simulink model "SqaureKF"  (Simulink 7.6)
settings: Solver=ode8  StartTime=0.0  StopTime=inf  FixedStep=0.01  RelTol=1e-3
libraries: aerolibanimutils x1, dspadpt3 x1, simulink x1
settings Model: Creator=Owen  LastModifiedBy=Owen

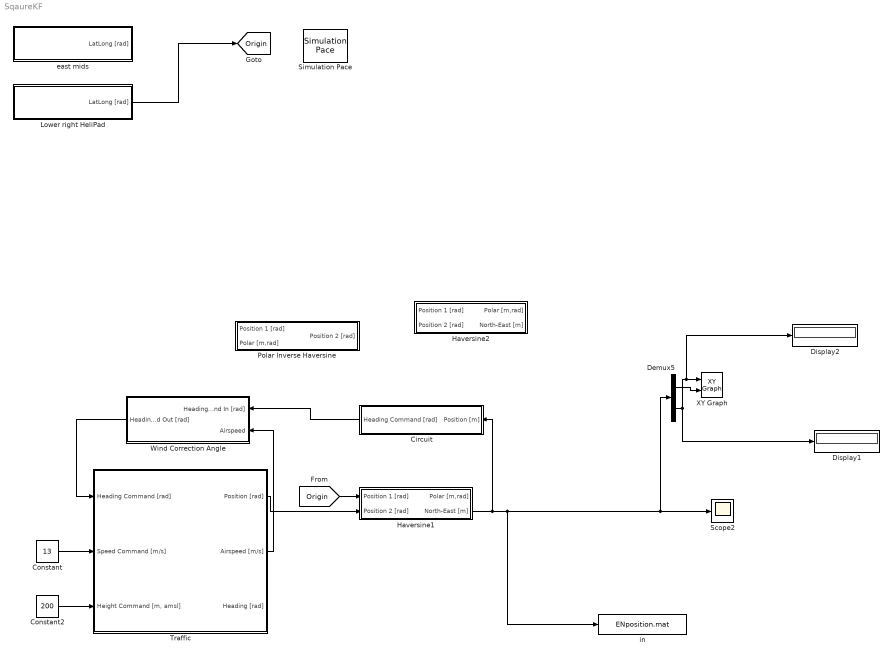
== system SqaureKF ==
  Circuit : Subsystem
  Constant : Constant  Value=13
  Constant2 : Constant  Value=200
  Demux5 : Demux  Outputs=2
  Display1 : Display
  Display2 : Display
  Haversine1 : Subsystem  mask{EARTH_RADIUS=6378100}
      mask prompts: EARTH_RADIUS "Radius of earth [m]"
  Haversine2 : Subsystem  mask{EARTH_RADIUS=6378100}
      mask prompts: EARTH_RADIUS "Radius of earth [m]"
  Lower right HeliPad : Subsystem  mask{LATITUDE=52.755938, LONGITUDE=-1.245055}
      mask prompts: LATITUDE "Latitude [decimal degrees]"; LONGITUDE "Longitude [decimal degrees]"
      mask Display:
      | fprintf('\n\n[%f, %f]',LATITUDE,LONGITUDE);
      | port_label('output',1,'LatLong [rad]');
  Polar Inverse Haversine : Subsystem  mask{EARTH_RADIUS=6378100}
      mask prompts: EARTH_RADIUS "Radius of earth [m]"
  Scope2 : Scope
      settings: TimeRange=100  YMin=-27.5  YMax=27.5  SaveName=UC  DataFormat=Array
  Simulation Pace : aerolibanimutils/Simulation Pace  SimulationPace=1  SleepMode=MATLAB Thread  OutputPaceError=off  SampleTime=1/10
      settings: AttributesFormatString=%<SimulationPace> sec/sec
  Traffic : Subsystem
  Wind Correction Angle : Subsystem  mask{WINDSPEED=9, WINDHEADING=260}
      mask prompts: WINDSPEED "Wind Speed [m/s]"; WINDHEADING "Wind Heading [deg]"
  XY Graph : simulink/Sinks/XY Graph  SystemSampleTime=-1  xmin=-300  xmax=300  ymin=-300  ymax=300  st=-1
  east mids : Subsystem  mask{LATITUDE=52.828961, LONGITUDE=-1.307569}
      mask prompts: LATITUDE "Latitude [decimal degrees]"; LONGITUDE "Longitude [decimal degrees]"
      mask Display:
      | fprintf('\n\n[%f, %f]',LATITUDE,LONGITUDE);
      | port_label('output',1,'LatLong [rad]');
  in : ToFile  Filename=ENposition.mat  SaveFormat=Timeseries
  tag scope: Origin=global
  wires:
  Constant/1 -> Traffic/2(Speed Command [m/s])
  Constant2/1 -> Traffic/3("Height Command [m, amsl]")
  Traffic/1(Position [rad]) -> Haversine1/2(Position 2 [rad])
  [Origin] -> Haversine1/1(Position 1 [rad])
  Haversine1/2(North-East [m]) -> Circuit/1(Position [m]), in/1, Scope2/1, Demux5/1
  Demux5/2 -> XY Graph/1, Display2/1, Display1/1
  Demux5/1 -> XY Graph/2
  Lower right HeliPad/1(LatLong [rad]) -> [Origin]
  Wind Correction Angle/1(Heading Command Out [rad]) -> Traffic/1(Heading Command [rad])
  Circuit/1(Heading Command [rad]) -> Wind Correction Angle/1(Heading Command In [rad])
  Traffic/2(Airspeed [m/s]) -> Wind Correction Angle/2(Airspeed)

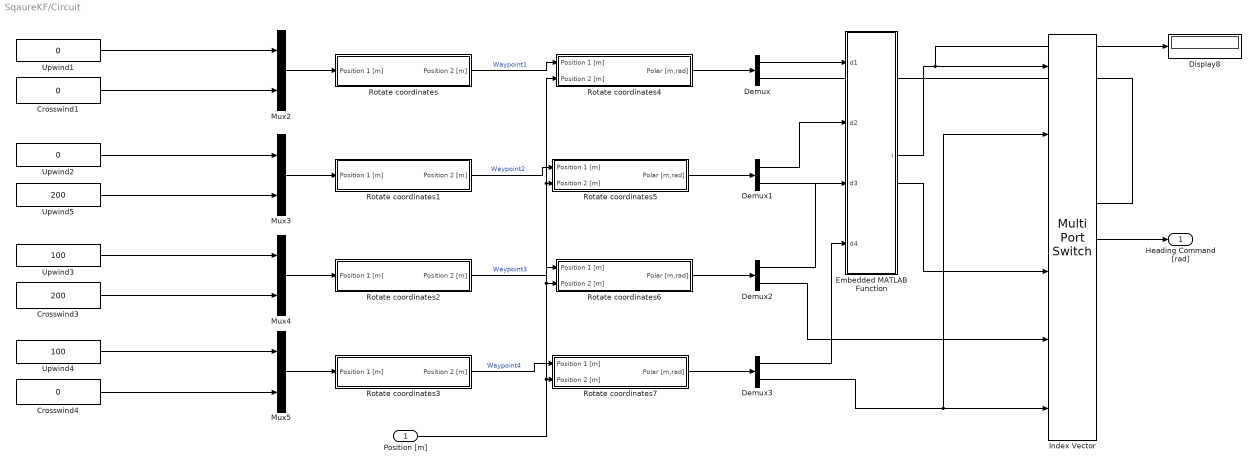
== system SqaureKF/Circuit ==
  Position [m] : Inport
  Crosswind1 : Constant  Value=0  VectorParams1D=off
  Crosswind3 : Constant  Value=200  VectorParams1D=off
  Crosswind4 : Constant  Value=0  VectorParams1D=off
  Demux{,1..3} (4 alike) : Demux  Outputs=2
  Display8 : Display
  Embedded MATLAB Function : Stateflow chart  TreatAsAtomicUnit=on
  Index Vector : MultiPortSwitch  DataPortOrder=Zero-based contiguous  Inputs=5  zeroidx=on
  Mux{2..5} (4 alike) : Mux  Inputs=2
  Rotate coordinates : Subsystem  mask{ANGLE=0, DIR=1}
      mask prompts: DIR "Direction"
  Rotate coordinates1 : Subsystem  mask{ANGLE=0, DIR=1}
      mask prompts: DIR "Direction"
  Rotate coordinates2 : Subsystem  mask{ANGLE=0, DIR=1}
      mask prompts: DIR "Direction"
  Rotate coordinates3 : Subsystem  mask{ANGLE=0, DIR=1}
      mask prompts: DIR "Direction"
  Rotate coordinates4 : Subsystem
  Rotate coordinates5 : Subsystem
  Rotate coordinates6 : Subsystem
  Rotate coordinates7 : Subsystem
  Upwind1 : Constant  Value=0
  Upwind2 : Constant  Value=0
  Upwind3 : Constant  Value=100
  Upwind4 : Constant  Value=100
  Upwind5 : Constant  Value=200
  Heading Command [rad] : Outport
  wires:
  Upwind1/1 -> Mux2/1
  Mux2/1 -> Rotate coordinates/1(Position 1 [m])
  Mux3/1 -> Rotate coordinates1/1(Position 1 [m])
  Crosswind3/1 -> Mux4/2
  Mux4/1 -> Rotate coordinates2/1(Position 1 [m])
  Upwind4/1 -> Mux5/1
  Crosswind4/1 -> Mux5/2
  Mux5/1 -> Rotate coordinates3/1(Position 1 [m])
  Rotate coordinates/1(Position 2 [m]) -> Rotate coordinates4/1(Position 1 [m])  "Waypoint1"
  Rotate coordinates1/1(Position 2 [m]) -> Rotate coordinates5/1(Position 1 [m])  "Waypoint2"
  Rotate coordinates2/1(Position 2 [m]) -> Rotate coordinates6/1(Position 1 [m])  "Waypoint3"
  Rotate coordinates3/1(Position 2 [m]) -> Rotate coordinates7/1(Position 1 [m])  "Waypoint4"
  Rotate coordinates4/1(Polar [m,rad]) -> Demux/1
  Rotate coordinates5/1(Polar [m,rad]) -> Demux1/1
  Rotate coordinates6/1(Polar [m,rad]) -> Demux2/1
  Rotate coordinates7/1(Polar [m,rad]) -> Demux3/1
  Demux/1 -> Embedded MATLAB Function/1(d1)
  Demux1/1 -> Embedded MATLAB Function/2(d2)
  Demux2/1 -> Embedded MATLAB Function/3(d3)
  Demux3/1 -> Embedded MATLAB Function/4(d4)
  Embedded MATLAB Function/1(i) -> Index Vector/1, Display8/1
  Position [m]/1 -> Rotate coordinates4/2(Position 2 [m]), Rotate coordinates5/2(Position 2 [m]), Rotate coordinates6/2(Position 2 [m]), Rotate coordinates7/2(Position 2 [m])
  Index Vector/1 -> Heading Command [rad]/1
  Demux3/2 -> Index Vector/6, Index Vector/2
  Demux2/2 -> Index Vector/5
  Demux1/2 -> Index Vector/4
  Demux/2 -> Index Vector/3
  Upwind2/1 -> Mux3/1
  Crosswind1/1 -> Mux2/2
  Upwind3/1 -> Mux4/1
  Upwind5/1 -> Mux3/2

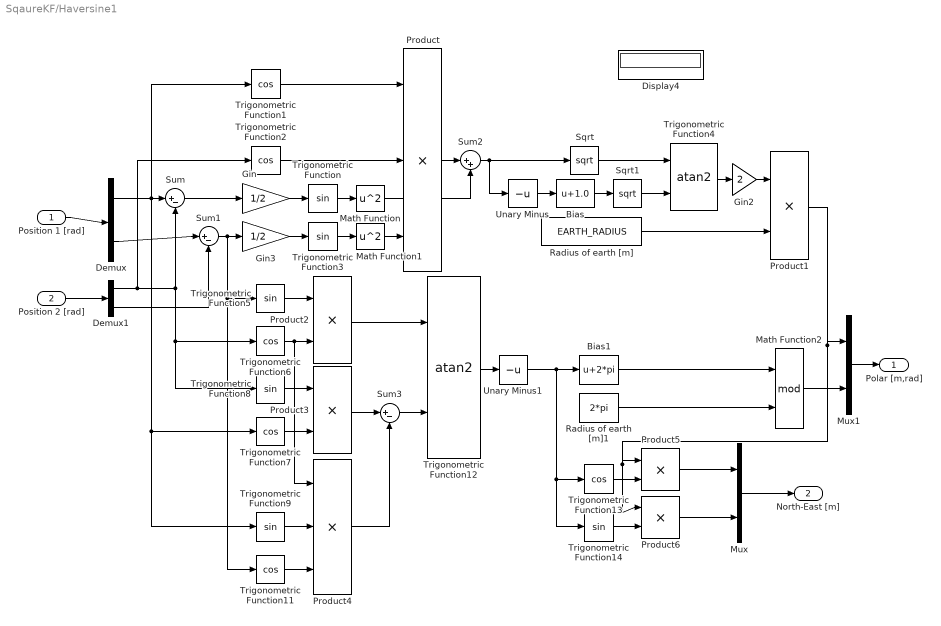
== system SqaureKF/Haversine1 ==
  Position 1 [rad] : Inport
  Position 2 [rad] : Inport  Port=2
  Bias : Bias  Bias=1.0
  Bias1 : Bias  Bias=2*pi
  Demux : Demux  Outputs=2
  Demux1 : Demux  Outputs=2
  Display4 : Display
  Gin : Gain  Gain=1/2
  Gin2 : Gain  Gain=2
  Gin3 : Gain  Gain=1/2
  Math Function : Math  Operator=square  SaturateOnIntegerOverflow=on
  Math Function1 : Math  Operator=square  SaturateOnIntegerOverflow=on
  Math Function2 : Math  Operator=mod  SaturateOnIntegerOverflow=on
  Mux : Mux  Inputs=2
  Mux1 : Mux  Inputs=2
  Product : Product  Inputs=3  RndMeth=Zero
  Product{1..3,5..6} (5 alike) : Product  RndMeth=Zero
  Product4 : Product  Inputs=3  RndMeth=Zero
  Radius of earth [m] : Constant  Value=EARTH_RADIUS
  Radius of earth [m]1 : Constant  Value=2*pi
  Sqrt : Sqrt  SaturateOnIntegerOverflow=on
  Sqrt1 : Sqrt  SaturateOnIntegerOverflow=on
  Sum : Sum  Inputs=|+-
  Sum1 : Sum  Inputs=|+-
  Sum2 : Sum  Inputs=|++
  Sum3 : Sum  Inputs=|+-
  Trigonometric Function{,3,5,8..9,14} (6 alike) : Trigonometry
  Trigonometric Function{1..2,6..7,11,13} (6 alike) : Trigonometry  Operator=cos
  Trigonometric Function12 : Trigonometry  Operator=atan2
  Trigonometric Function4 : Trigonometry  Operator=atan2
  Unary Minus : UnaryMinus
  Unary Minus1 : UnaryMinus
  Polar [m,rad] : Outport
  North-East [m] : Outport  Port=2
  wires:
  Unary Minus1/1 -> Trigonometric Function13/1, Trigonometric Function14/1, Bias1/1
  Bias1/1 -> Math Function2/1
  Position 2 [rad]/1 -> Demux1/1
  Position 1 [rad]/1 -> Demux/1
  Sum3/1 -> Trigonometric Function12/2
  Product2/1 -> Trigonometric Function12/1
  Sqrt1/1 -> Trigonometric Function4/2
  Sqrt/1 -> Trigonometric Function4/1
  Gin2/1 -> Product1/1
  Trigonometric Function4/1 -> Gin2/1
  Demux/1 -> Trigonometric Function1/1, Sum/1, Trigonometric Function7/1, Trigonometric Function9/1
  Demux/2 -> Sum1/1
  Demux1/1 -> Trigonometric Function2/1, Trigonometric Function8/1, Trigonometric Function6/1, Sum/2
  Demux1/2 -> Sum1/2
  Sum/1 -> Gin/1
  Gin/1 -> Trigonometric Function/1
  Trigonometric Function/1 -> Math Function/1
  Gin3/1 -> Trigonometric Function3/1
  Trigonometric Function3/1 -> Math Function1/1
  Sum1/1 -> Gin3/1, Trigonometric Function5/1, Trigonometric Function11/1
  Trigonometric Function1/1 -> Product/1
  Trigonometric Function2/1 -> Product/2
  Math Function1/1 -> Product/3
  Product/1 -> Sum2/1
  Math Function/1 -> Sum2/2
  Sum2/1 -> Sqrt/1, Unary Minus/1
  Unary Minus/1 -> Bias/1
  Bias/1 -> Sqrt1/1
  Product1/1 -> Product5/1, Product6/1, Mux1/1
  Radius of earth [m]/1 -> Product1/2
  Trigonometric Function5/1 -> Product2/1
  Trigonometric Function6/1 -> Product4/1, Product2/2
  Trigonometric Function8/1 -> Product3/1
  Trigonometric Function7/1 -> Product3/2
  Trigonometric Function9/1 -> Product4/2
  Trigonometric Function11/1 -> Product4/3
  Product3/1 -> Sum3/1
  Product4/1 -> Sum3/2
  Trigonometric Function12/1 -> Unary Minus1/1
  Mux/1 -> North-East [m]/1
  Trigonometric Function13/1 -> Product5/2
  Product5/1 -> Mux/1
  Product6/1 -> Mux/2
  Trigonometric Function14/1 -> Product6/2
  Math Function2/1 -> Mux1/2
  Radius of earth [m]1/1 -> Math Function2/2
  Mux1/1 -> Polar [m,rad]/1

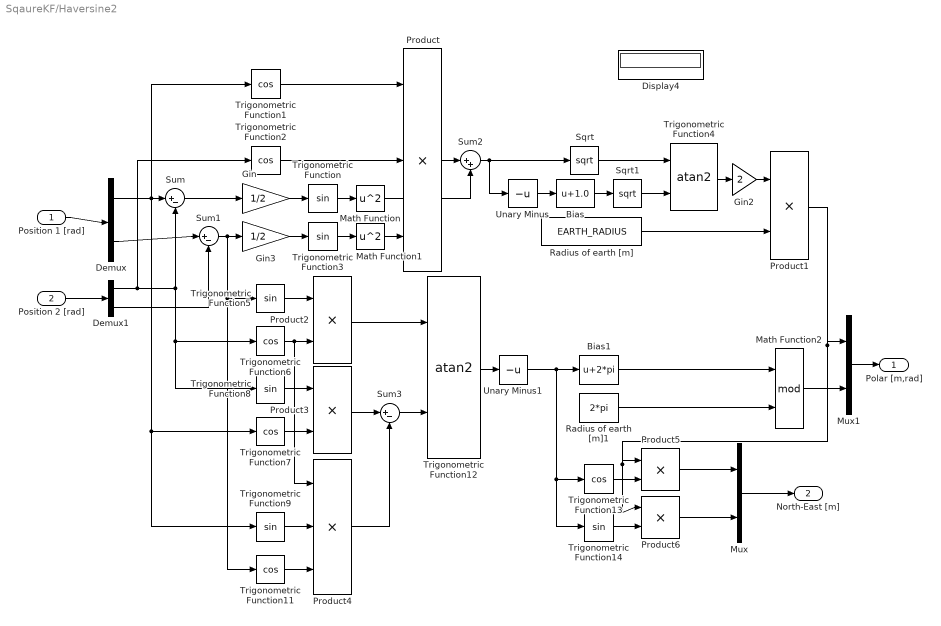
== system SqaureKF/Haversine2 ==
  Position 1 [rad] : Inport
  Position 2 [rad] : Inport  Port=2
  Bias : Bias  Bias=1.0
  Bias1 : Bias  Bias=2*pi
  Demux : Demux  Outputs=2
  Demux1 : Demux  Outputs=2
  Display4 : Display
  Gin : Gain  Gain=1/2
  Gin2 : Gain  Gain=2
  Gin3 : Gain  Gain=1/2
  Math Function : Math  Operator=square  SaturateOnIntegerOverflow=on
  Math Function1 : Math  Operator=square  SaturateOnIntegerOverflow=on
  Math Function2 : Math  Operator=mod  SaturateOnIntegerOverflow=on
  Mux : Mux  Inputs=2
  Mux1 : Mux  Inputs=2
  Product : Product  Inputs=3  RndMeth=Zero
  Product{1..3,5..6} (5 alike) : Product  RndMeth=Zero
  Product4 : Product  Inputs=3  RndMeth=Zero
  Radius of earth [m] : Constant  Value=EARTH_RADIUS
  Radius of earth [m]1 : Constant  Value=2*pi
  Sqrt : Sqrt  SaturateOnIntegerOverflow=on
  Sqrt1 : Sqrt  SaturateOnIntegerOverflow=on
  Sum : Sum  Inputs=|+-
  Sum1 : Sum  Inputs=|+-
  Sum2 : Sum  Inputs=|++
  Sum3 : Sum  Inputs=|+-
  Trigonometric Function{,3,5,8..9,14} (6 alike) : Trigonometry
  Trigonometric Function{1..2,6..7,11,13} (6 alike) : Trigonometry  Operator=cos
  Trigonometric Function12 : Trigonometry  Operator=atan2
  Trigonometric Function4 : Trigonometry  Operator=atan2
  Unary Minus : UnaryMinus
  Unary Minus1 : UnaryMinus
  Polar [m,rad] : Outport
  North-East [m] : Outport  Port=2
  wires:
  Unary Minus1/1 -> Trigonometric Function13/1, Trigonometric Function14/1, Bias1/1
  Bias1/1 -> Math Function2/1
  Position 2 [rad]/1 -> Demux1/1
  Position 1 [rad]/1 -> Demux/1
  Sum3/1 -> Trigonometric Function12/2
  Product2/1 -> Trigonometric Function12/1
  Sqrt1/1 -> Trigonometric Function4/2
  Sqrt/1 -> Trigonometric Function4/1
  Gin2/1 -> Product1/1
  Trigonometric Function4/1 -> Gin2/1
  Demux/1 -> Trigonometric Function1/1, Sum/1, Trigonometric Function7/1, Trigonometric Function9/1
  Demux/2 -> Sum1/1
  Demux1/1 -> Trigonometric Function2/1, Trigonometric Function8/1, Trigonometric Function6/1, Sum/2
  Demux1/2 -> Sum1/2
  Sum/1 -> Gin/1
  Gin/1 -> Trigonometric Function/1
  Trigonometric Function/1 -> Math Function/1
  Gin3/1 -> Trigonometric Function3/1
  Trigonometric Function3/1 -> Math Function1/1
  Sum1/1 -> Gin3/1, Trigonometric Function5/1, Trigonometric Function11/1
  Trigonometric Function1/1 -> Product/1
  Trigonometric Function2/1 -> Product/2
  Math Function1/1 -> Product/3
  Product/1 -> Sum2/1
  Math Function/1 -> Sum2/2
  Sum2/1 -> Sqrt/1, Unary Minus/1
  Unary Minus/1 -> Bias/1
  Bias/1 -> Sqrt1/1
  Product1/1 -> Product5/1, Product6/1, Mux1/1
  Radius of earth [m]/1 -> Product1/2
  Trigonometric Function5/1 -> Product2/1
  Trigonometric Function6/1 -> Product4/1, Product2/2
  Trigonometric Function8/1 -> Product3/1
  Trigonometric Function7/1 -> Product3/2
  Trigonometric Function9/1 -> Product4/2
  Trigonometric Function11/1 -> Product4/3
  Product3/1 -> Sum3/1
  Product4/1 -> Sum3/2
  Trigonometric Function12/1 -> Unary Minus1/1
  Mux/1 -> North-East [m]/1
  Trigonometric Function13/1 -> Product5/2
  Product5/1 -> Mux/1
  Product6/1 -> Mux/2
  Trigonometric Function14/1 -> Product6/2
  Math Function2/1 -> Mux1/2
  Radius of earth [m]1/1 -> Math Function2/2
  Mux1/1 -> Polar [m,rad]/1

== system SqaureKF/Lower right HeliPad ==
  Gin : Gain  Gain=pi/180
  Gin1 : Gain  Gain=pi/180
  Mux : Mux  Inputs=2
  Radius of earth [m]1 : Constant  Value=LONGITUDE
  Radius of earth [m]2 : Constant  Value=LATITUDE
  LatLong [rad] : Outport
  wires:
  Radius of earth [m]2/1 -> Gin/1
  Radius of earth [m]1/1 -> Gin1/1
  Mux/1 -> LatLong [rad]/1
  Gin/1 -> Mux/1
  Gin1/1 -> Mux/2

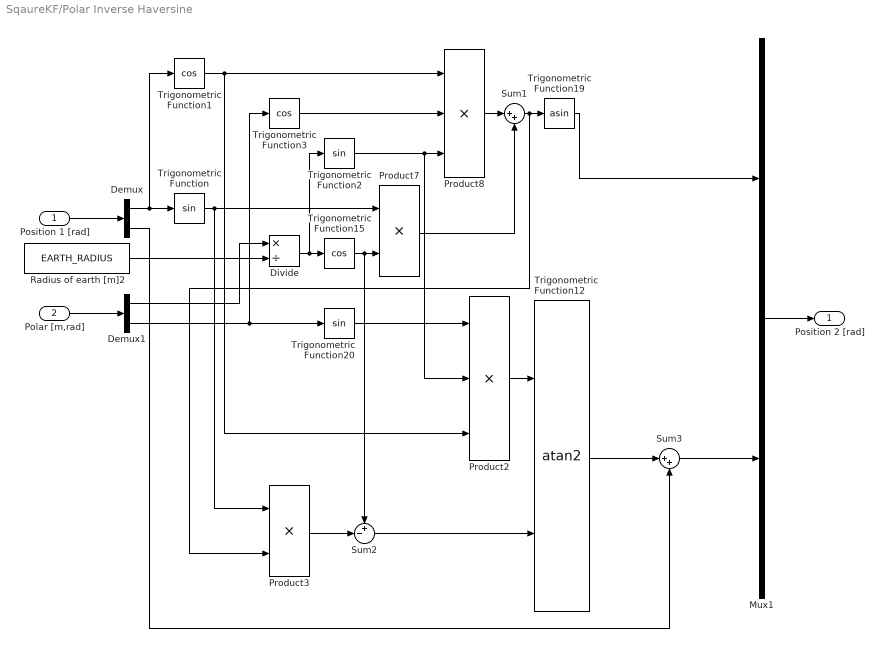
== system SqaureKF/Polar Inverse Haversine ==
  Position 1 [rad] : Inport
  Polar [m,rad] : Inport  Port=2
  Demux : Demux  Outputs=2
  Demux1 : Demux  Outputs=2
  Divide : Product  Inputs=*/
  Mux1 : Mux  Inputs=2
  Product2 : Product  Inputs=3  RndMeth=Zero
  Product3 : Product  RndMeth=Zero
  Product7 : Product  RndMeth=Zero
  Product8 : Product  Inputs=3  RndMeth=Zero
  Radius of earth [m]2 : Constant  Value=EARTH_RADIUS
  Sum1 : Sum  Inputs=|++
  Sum2 : Sum  Inputs=+-|
  Sum3 : Sum  Inputs=|++
  Trigonometric Function : Trigonometry
  Trigonometric Function1 : Trigonometry  Operator=cos
  Trigonometric Function12 : Trigonometry  Operator=atan2
  Trigonometric Function15 : Trigonometry  Operator=cos
  Trigonometric Function19 : Trigonometry  Operator=asin
  Trigonometric Function2 : Trigonometry
  Trigonometric Function20 : Trigonometry
  Trigonometric Function3 : Trigonometry  Operator=cos
  Position 2 [rad] : Outport
  wires:
  Position 1 [rad]/1 -> Demux/1
  Polar [m,rad]/1 -> Demux1/1
  Demux/1 -> Trigonometric Function/1, Trigonometric Function1/1
  Radius of earth [m]2/1 -> Divide/2
  Demux1/1 -> Divide/1
  Divide/1 -> Trigonometric Function2/1, Trigonometric Function15/1
  Trigonometric Function15/1 -> Product7/2, Sum2/1
  Trigonometric Function/1 -> Product7/1, Product3/1
  Demux1/2 -> Trigonometric Function3/1, Trigonometric Function20/1
  Trigonometric Function2/1 -> Product8/3, Product2/2
  Trigonometric Function3/1 -> Product8/2
  Trigonometric Function1/1 -> Product8/1, Product2/3
  Product8/1 -> Sum1/1
  Product7/1 -> Sum1/2
  Sum1/1 -> Product3/2, Trigonometric Function19/1
  Demux/2 -> Sum3/2
  Trigonometric Function20/1 -> Product2/1
  Product2/1 -> Trigonometric Function12/1
  Product3/1 -> Sum2/2
  Trigonometric Function19/1 -> Mux1/1
  Sum2/1 -> Trigonometric Function12/2
  Trigonometric Function12/1 -> Sum3/1
  Sum3/1 -> Mux1/2
  Mux1/1 -> Position 2 [rad]/1

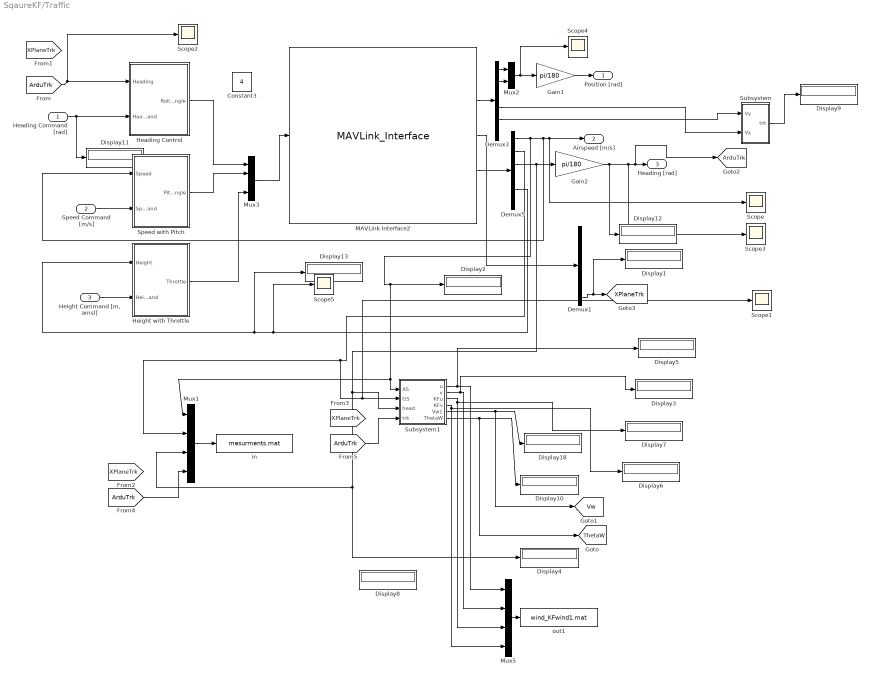
== system SqaureKF/Traffic ==
  Heading Command [rad] : Inport
  Speed Command [m/s] : Inport  Port=2
  "Height Command [m, amsl]" : Inport  Port=3
  Constant3 : Constant  Value=4
  Demux1 : Demux  Outputs=5
  Demux3 : Demux  Outputs=6
  Demux5 : Demux  Outputs=6
  Display{1..13,18} (14 alike) : Display
  Gain1 : Gain  Gain=pi/180
  Gain2 : Gain  Gain=pi/180
  Heading Control : Subsystem
  Height with Throttle : Subsystem
  MAVLink Interface2 : S-Function  FunctionName=MAVLink_Interface  Parameters=COM_Port,Baud_Rate,IP_ADDRESS,IP_PORT,SYS_ID,COMP_ID,COMP_TARG,MSG_INPUT,MSG_OUTPUT  EnableBusSupport=off  mask{COM_Port='COM6', Baud_Rate=115200, IP_ADDRESS='', IP_PORT=5013, SYS_ID=255, COMP_ID=0, COMP_TARG='/aircraft/LU-WOTB/APM', HEART_BEAT=off, ATTITUDE_OUT=on, RAW_IMU=off, POSITION_OUT=on, POSITION_OUT2=on, VFR_HUD=on, RC_SCALED=off, SERVO_OUT_RAW=off, SYS_STATUS=on, SET_MODE=off, DATA_STREAM=off, ATTITUDE_COMMAND=on, RC_OVERRIDE=off, ATTITUDE_IN=off, GPS_RAW_IN=off, VFR_HUD_IN=off}
      mask prompts: COM_Port "COM Port"; Baud_Rate "Baud Rate"; IP_ADDRESS "IP Address"; IP_PORT "Port"; SYS_ID "System ID"; COMP_ID "Component ID"; COMP_TARG "Target Component"; HEART_BEAT "Heartbeat"; ATTITUDE_OUT "Attitude"; RAW_IMU "Raw IMU"; POSITION_OUT "Global Position"; POSITION_OUT2 "Global Position 2"; VFR_HUD "VFR HUD"; RC_SCALED "Scaled RC Channels"; SERVO_OUT_RAW "Raw Servo Positions"; SYS_STATUS "System Status"; SET_MODE "Mode"; DATA_STREAM "Datastream Request"; ATTITUDE_COMMAND "Attitude Command"; RC_OVERRIDE "RC Override"; ATTITUDE_IN "Attitude (HIL)"; GPS_RAW_IN "Raw GPS (HIL)"; VFR_HUD_IN "VFR HUD (HIL)"
      mask init:
      | MSG_ID_NUM_INPUT = [uint8(11) uint8(66) uint8(70) uint8(55) uint8(30) uint8(32) uint8(73)];
      | MSG_ID_NAME_INPUT = [SET_MODE DATA_STREAM RC_OVERRIDE ATTITUDE_COMMAND ATTITUDE_IN GPS_RAW_IN VFR_HUD_IN];
      | 
      | MSG_ID_NUM_OUTPUT = [uint8(0) uint8(30) uint8(28) uint8(73) uint8(32) uint8(74) uint8(36) uint8(37) uint8(34)];
      | MSG_ID_NAME_OUTPUT = [HEART_BEAT ATTITUDE_OUT RAW_IMU VFR_HUD POSITION_OUT2 POSITION_OUT RC_SCALED SERVO_OUT_RAW SYS_STATUS];
      | 
      | idx_input = find(MSG_ID_NAME_INPUT);
      | MSG_INPUT = MSG_ID_NUM_INPUT(idx_input);
      | 
      | idx_output = find(MSG_ID_NAME_OUTPUT);
      | MSG_OUTPUT = MSG_ID_NUM_OUTPUT(idx_output);
      mask TabNameString: Connection,Connection,Connection,Connection,MAVLink,MAVLink,MAVLink,Outputs,Outputs,Outputs,Outputs,Outputs,Outputs,Outputs,Outputs,Outputs,Inputs,Inputs,Inputs,Inputs,Inputs,Inputs,Inputs
      mask Display:
      | %Label block
      | 
      | if (~strcmp(COM_Port, ''))
      | fprintf('MAVLink Serial\n%s\n%dbps', COM_Port,  Baud_Rate)
      | end
      | if (~strcmp(IP_ADDRESS, ''))
      | fprintf('MAVLink TCP\n%s:%d', IP_ADDRESS,  IP_PORT)
      | end
      | fprintf('\n\n\n\n\n%d:%d\n%s', SYS_ID, COMP_ID, COMP_TARG)
      | 
      | 
      | %Label input ports
      | 
      | in = 1;
      | if (SET_MODE == 1)
      |     port_label('input', in, 'Mode');
      |     in = in + 1;
      | end
      | if (DATA_STREAM == 1)
      |     port_label('input', in, 'Datastream Request');
      |     in = in + 1;
      | end
      | if (ATTITUDE_COMMAND == 1)
      |     port_label('input', in, 'Attitude Command');
      |     in = in + 1;
      | end
      | if (ATTITUDE_IN == 1)
      |     port_label('input', in, 'Attitude (HIL)');
      |     in = in + 1;
      | end
      | if (GPS_RAW_IN == 1)
      |     port_label('input', in, 'Raw GPS (HIL)');
      |     in = in + 1;
      | end
      | if (VFR_HUD_IN == 1)
      |     port_label('input', in, 'VFR HUD (HIL)');
      |     in = in + 1;
      | end
      | 
      | %Label output ports
      | 
      | out = 1;
      | if (HEART_BEAT == 1)
      |     port_label('output', out, 'Heartbeat');
      |     out = out + 1;
      | end
      | if (ATTITUDE_OUT == 1)
      |     port_label('output', out, 'Attitude');
      |     out = out + 1;
      | end
      | if (RAW_IMU == 1)
      |     port_label('output', out, 'Raw IMU');
      |     out = out + 1;
      | end
      | if (POSITION_OUT == 1)
      |     port_label('output', out, 'Global Position');
      |     out = out + 1;
      | end
      | if (POSITION_OUT2 == 1)
      |     port_label('output', out, 'Global Position 2');
      |     out = out + 1;
      | end
      | if (VFR_HUD == 1)
      |     port_label('output', out, 'VFR HUD');
      |     out = out + 1;
      | end
      | if (RC_SCALED == 1)
      |     port_label('output', out, 'Scaled RC Channels');
      |     out = out + 1;
      | end
      | if (SERVO_OUT_RAW == 1)
      |     port_label('output', out, 'Raw Servo Output');
      |     out = out + 1;
      | end
      | if (SYS_STATUS == 1)
      |     port_label('output', out, 'System Status');
      |     out = out + 1;
      | end
  Mux1 : Mux
  Mux2 : Mux  Inputs=2
  Mux3 : Mux
  Mux5 : Mux
  Scope{,1..5} (6 alike) : Scope
      Scope settings: YMin=0  YMax=8
      Scope2 settings: YMin=200  YMax=270  SaveName=ScopeData2
      Scope3 settings: YMin=2.25  SaveName=ScopeData3
      Scope4 settings: YMin=-2.5  YMax=55  SaveName=ScopeData4
      Scope5 settings: YMin=189.5  YMax=195  SaveName=ScopeData5
  Speed with Pitch : Subsystem
  Subsystem : Subsystem
  Subsystem1 : Subsystem
  in : ToFile  Filename=mesurments.mat  SaveFormat=Timeseries
  out1 : ToFile  Filename=wind_KFwind1.mat  SaveFormat=Timeseries
  Position [rad] : Outport
  Airspeed [m/s] : Outport  Port=2
  Heading [rad] : Outport  Port=3
  tag scope: ArduTrk=global, ThetaW=global, Vw=global, XPlaneTrk=global
  wires:
  Demux3/1 -> Mux2/1
  Demux3/2 -> Mux2/2
  Mux2/1 -> Gain1/1, Scope4/1
  MAVLink Interface2/2 -> Demux3/1
  MAVLink Interface2/4 -> Demux5/1
  Demux5/1 -> Speed with Pitch/1(Speed), Airspeed [m/s]/1, Scope/1, Display2/1, Subsystem1/1(AS), Mux1/1
  Demux5/5 -> Scope5/1, Height with Throttle/1(Height), Display13/1
  Demux5/3 -> Gain2/1, Subsystem1/3(head), Display4/1, Mux1/3
  Gain2/1 -> Display12/1, Scope3/1, Heading [rad]/1, [ArduTrk]
  Heading Command [rad]/1 -> Heading Control/2(Heading Command), Display11/1
  Speed Command [m/s]/1 -> Speed with Pitch/2(Speed  Command)
  "Height Command [m, amsl]"/1 -> Height with Throttle/2(Height  Command)
  Gain1/1 -> Position [rad]/1
  MAVLink Interface2/3 -> Demux1/1
  Demux5/2 -> Mux1/2, Subsystem1/2(GS), Scope1/1
  Mux5/1 -> out1/1
  Subsystem1/1(u) -> Mux5/1, Display5/1
  Subsystem1/2(v) -> Mux5/2, Display3/1
  Subsystem1/3(KFu) -> Mux5/3, Display7/1
  Subsystem1/4(KFv) -> Mux5/4, Display6/1
  Subsystem1/5(Vw1) -> Display18/1, [Vw]
  Subsystem1/6(ThetaW) -> Display10/1, [ThetaW]
  Mux1/1 -> in/1
  Demux3/5 -> Subsystem/1(Vy)
  Heading Control/1(Roll Angle) -> Mux3/1
  Speed with Pitch/1(Pitch Angle) -> Mux3/2
  Height with Throttle/1(Throttle) -> Mux3/4
  Mux3/1 -> MAVLink Interface2/1
  Demux3/4 -> Subsystem/2(Vx)
  Subsystem/1(trk) -> Display9/1
  Demux1/5 -> [XPlaneTrk], Display1/1
  [ArduTrk] -> Mux1/4
  [ArduTrk] -> Scope2/1, Heading Control/1(Heading)
  [ArduTrk] -> Subsystem1/4(trk)

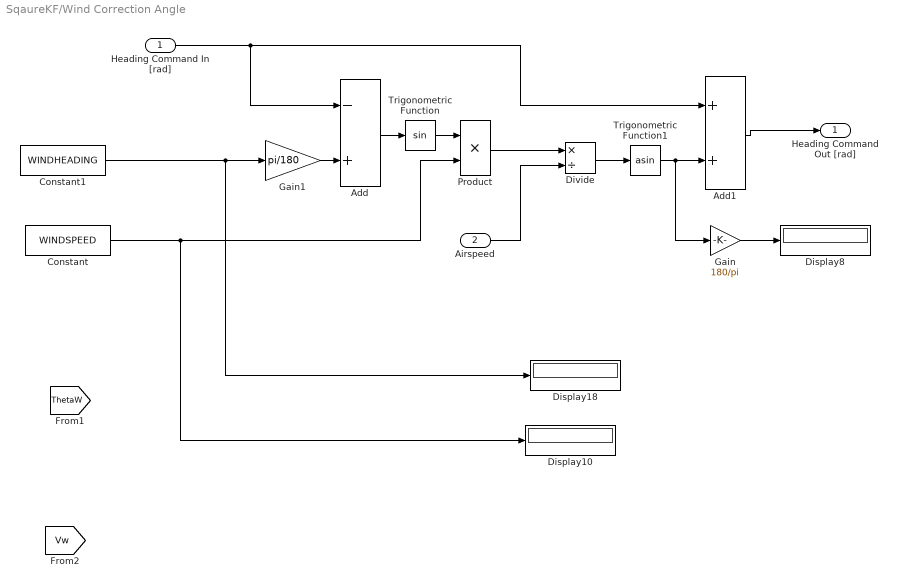
== system SqaureKF/Wind Correction Angle ==
  Heading Command In [rad] : Inport
  Airspeed : Inport  Port=2
  Add : Sum  Inputs=-+
  Add1 : Sum
  Constant : Constant  Value=WINDSPEED
  Constant1 : Constant  Value=WINDHEADING
  Display10 : Display
  Display18 : Display
  Display8 : Display
  Divide : Product  Inputs=*/
  Gain : Gain  Gain=180/pi
  Gain1 : Gain  Gain=pi/180
  Product : Product  RndMeth=Zero
  Trigonometric Function : Trigonometry
  Trigonometric Function1 : Trigonometry  Operator=asin
  Heading Command Out [rad] : Outport
  wires:
  Gain/1 -> Display8/1
  Gain1/1 -> Add/2
  Add1/1 -> Heading Command Out [rad]/1
  Trigonometric Function1/1 -> Gain/1, Add1/2
  Divide/1 -> Trigonometric Function1/1
  Airspeed/1 -> Divide/2
  Product/1 -> Divide/1
  Trigonometric Function/1 -> Product/1
  Add/1 -> Trigonometric Function/1
  Heading Command In [rad]/1 -> Add1/1, Add/1
  Constant/1 -> Product/2, Display10/1
  Constant1/1 -> Gain1/1, Display18/1

== system SqaureKF/east mids ==
  Gin : Gain  Gain=pi/180
  Gin1 : Gain  Gain=pi/180
  Mux : Mux  Inputs=2
  Radius of earth [m]1 : Constant  Value=LONGITUDE
  Radius of earth [m]2 : Constant  Value=LATITUDE
  LatLong [rad] : Outport
  wires:
  Radius of earth [m]2/1 -> Gin/1
  Radius of earth [m]1/1 -> Gin1/1
  Mux/1 -> LatLong [rad]/1
  Gin/1 -> Mux/1
  Gin1/1 -> Mux/2

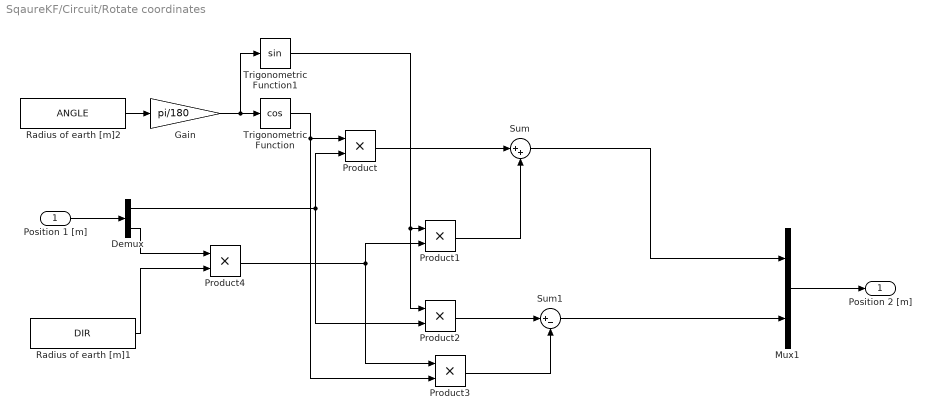
== system SqaureKF/Circuit/Rotate coordinates ==
  Position 1 [m] : Inport
  Demux : Demux  Outputs=2
  Gain : Gain  Gain=pi/180
  Mux1 : Mux  Inputs=2
  Product{,1..4} (5 alike) : Product  RndMeth=Zero
  Radius of earth [m]1 : Constant  Value=DIR
  Radius of earth [m]2 : Constant  Value=ANGLE
  Sum : Sum  Inputs=|++
  Sum1 : Sum  Inputs=|+-
  Trigonometric Function : Trigonometry  Operator=cos
  Trigonometric Function1 : Trigonometry
  Position 2 [m] : Outport
  wires:
  Mux1/1 -> Position 2 [m]/1
  Position 1 [m]/1 -> Demux/1
  Radius of earth [m]2/1 -> Gain/1
  Trigonometric Function/1 -> Product/1, Product3/2
  Demux/1 -> Product/2, Product2/2
  Trigonometric Function1/1 -> Product1/1, Product2/1
  Product/1 -> Sum/1
  Product1/1 -> Sum/2
  Sum/1 -> Mux1/1
  Product2/1 -> Sum1/1
  Product3/1 -> Sum1/2
  Sum1/1 -> Mux1/2
  Product4/1 -> Product3/1, Product1/2
  Demux/2 -> Product4/1
  Radius of earth [m]1/1 -> Product4/2
  Gain/1 -> Trigonometric Function/1, Trigonometric Function1/1

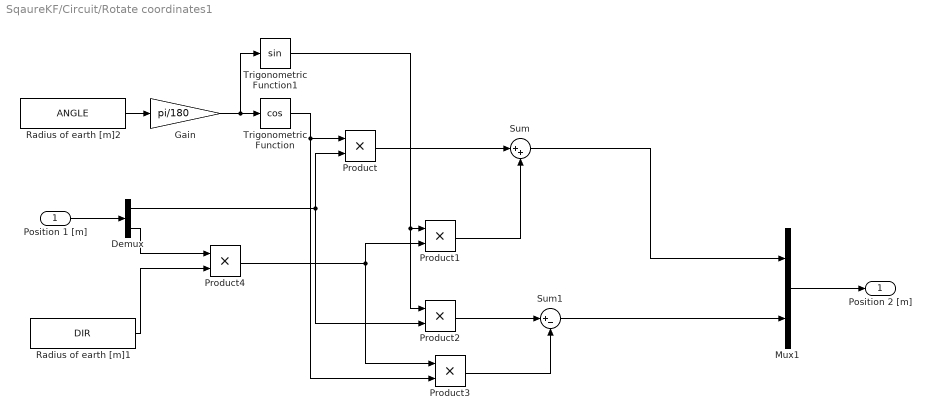
== system SqaureKF/Circuit/Rotate coordinates1 ==
  Position 1 [m] : Inport
  Demux : Demux  Outputs=2
  Gain : Gain  Gain=pi/180
  Mux1 : Mux  Inputs=2
  Product{,1..4} (5 alike) : Product  RndMeth=Zero
  Radius of earth [m]1 : Constant  Value=DIR
  Radius of earth [m]2 : Constant  Value=ANGLE
  Sum : Sum  Inputs=|++
  Sum1 : Sum  Inputs=|+-
  Trigonometric Function : Trigonometry  Operator=cos
  Trigonometric Function1 : Trigonometry
  Position 2 [m] : Outport
  wires:
  Gain/1 -> Trigonometric Function1/1, Trigonometric Function/1
  Radius of earth [m]1/1 -> Product4/2
  Demux/2 -> Product4/1
  Product4/1 -> Product1/2, Product3/1
  Sum1/1 -> Mux1/2
  Product3/1 -> Sum1/2
  Product2/1 -> Sum1/1
  Sum/1 -> Mux1/1
  Product1/1 -> Sum/2
  Product/1 -> Sum/1
  Trigonometric Function1/1 -> Product2/1, Product1/1
  Demux/1 -> Product2/2, Product/2
  Trigonometric Function/1 -> Product3/2, Product/1
  Radius of earth [m]2/1 -> Gain/1
  Position 1 [m]/1 -> Demux/1
  Mux1/1 -> Position 2 [m]/1

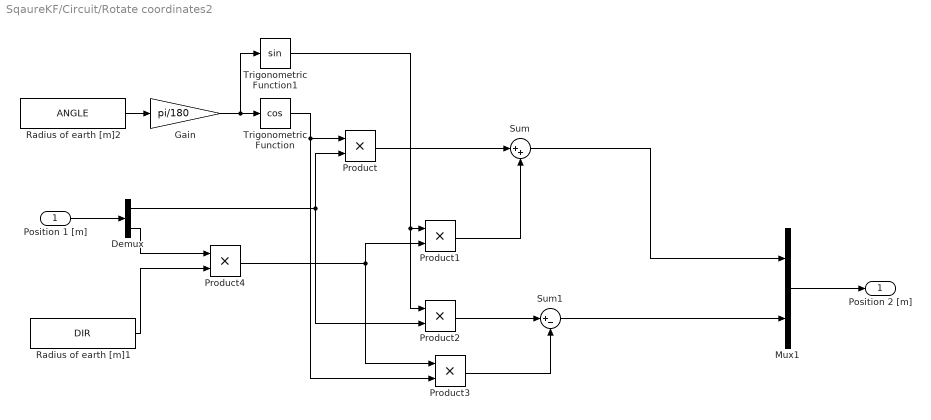
== system SqaureKF/Circuit/Rotate coordinates2 ==
  Position 1 [m] : Inport
  Demux : Demux  Outputs=2
  Gain : Gain  Gain=pi/180
  Mux1 : Mux  Inputs=2
  Product{,1..4} (5 alike) : Product  RndMeth=Zero
  Radius of earth [m]1 : Constant  Value=DIR
  Radius of earth [m]2 : Constant  Value=ANGLE
  Sum : Sum  Inputs=|++
  Sum1 : Sum  Inputs=|+-
  Trigonometric Function : Trigonometry  Operator=cos
  Trigonometric Function1 : Trigonometry
  Position 2 [m] : Outport
  wires:
  Mux1/1 -> Position 2 [m]/1
  Position 1 [m]/1 -> Demux/1
  Radius of earth [m]2/1 -> Gain/1
  Trigonometric Function/1 -> Product/1, Product3/2
  Demux/1 -> Product/2, Product2/2
  Trigonometric Function1/1 -> Product1/1, Product2/1
  Product/1 -> Sum/1
  Product1/1 -> Sum/2
  Sum/1 -> Mux1/1
  Product2/1 -> Sum1/1
  Product3/1 -> Sum1/2
  Sum1/1 -> Mux1/2
  Product4/1 -> Product3/1, Product1/2
  Demux/2 -> Product4/1
  Radius of earth [m]1/1 -> Product4/2
  Gain/1 -> Trigonometric Function/1, Trigonometric Function1/1

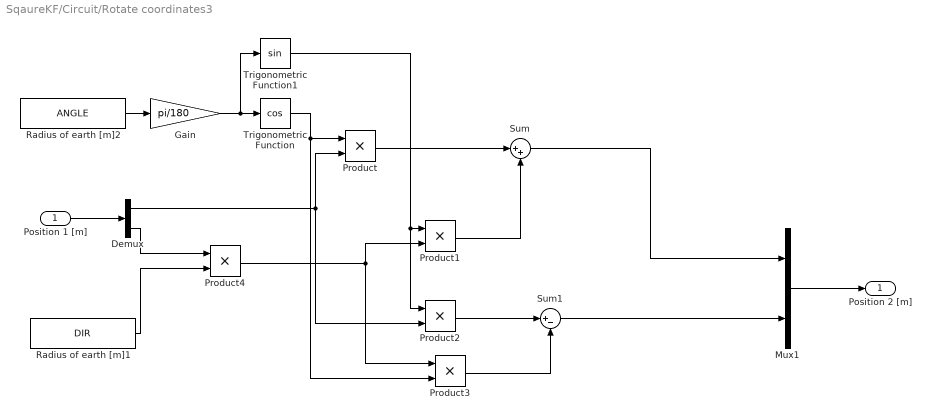
== system SqaureKF/Circuit/Rotate coordinates3 ==
  Position 1 [m] : Inport
  Demux : Demux  Outputs=2
  Gain : Gain  Gain=pi/180
  Mux1 : Mux  Inputs=2
  Product{,1..4} (5 alike) : Product  RndMeth=Zero
  Radius of earth [m]1 : Constant  Value=DIR
  Radius of earth [m]2 : Constant  Value=ANGLE
  Sum : Sum  Inputs=|++
  Sum1 : Sum  Inputs=|+-
  Trigonometric Function : Trigonometry  Operator=cos
  Trigonometric Function1 : Trigonometry
  Position 2 [m] : Outport
  wires:
  Gain/1 -> Trigonometric Function1/1, Trigonometric Function/1
  Radius of earth [m]1/1 -> Product4/2
  Demux/2 -> Product4/1
  Product4/1 -> Product1/2, Product3/1
  Sum1/1 -> Mux1/2
  Product3/1 -> Sum1/2
  Product2/1 -> Sum1/1
  Sum/1 -> Mux1/1
  Product1/1 -> Sum/2
  Product/1 -> Sum/1
  Trigonometric Function1/1 -> Product2/1, Product1/1
  Demux/1 -> Product2/2, Product/2
  Trigonometric Function/1 -> Product3/2, Product/1
  Radius of earth [m]2/1 -> Gain/1
  Position 1 [m]/1 -> Demux/1
  Mux1/1 -> Position 2 [m]/1

== system SqaureKF/Circuit/Rotate coordinates4 ==
  Position 1 [m] : Inport
  Position 2 [m] : Inport  Port=2
  Add : Sum
  Add1 : Sum  Inputs=+-
  Bias : Bias  Bias=2*pi
  Constant : Constant  Value=2*pi
  Demux : Demux  Outputs=2
  Math Function : Math  Operator=square  SaturateOnIntegerOverflow=on
  Math Function1 : Math  Operator=square  SaturateOnIntegerOverflow=on
  Math Function2 : Math  Operator=mod  SaturateOnIntegerOverflow=on
  Mux1 : Mux  Inputs=2
  Sqrt : Sqrt  SaturateOnIntegerOverflow=on
  Trigonometric Function : Trigonometry  Operator=atan2
  Polar [m,rad] : Outport
  wires:
  Mux1/1 -> Polar [m,rad]/1
  Add/1 -> Sqrt/1
  Math Function/1 -> Add/1
  Math Function1/1 -> Add/2
  Demux/1 -> Math Function/1, Trigonometric Function/2
  Demux/2 -> Math Function1/1, Trigonometric Function/1
  Sqrt/1 -> Mux1/1
  Trigonometric Function/1 -> Bias/1
  Bias/1 -> Math Function2/1
  Math Function2/1 -> Mux1/2
  Constant/1 -> Math Function2/2
  Position 1 [m]/1 -> Add1/1
  Position 2 [m]/1 -> Add1/2
  Add1/1 -> Demux/1

== system SqaureKF/Circuit/Rotate coordinates5 ==
  Position 1 [m] : Inport
  Position 2 [m] : Inport  Port=2
  Add : Sum
  Add1 : Sum  Inputs=+-
  Bias : Bias  Bias=2*pi
  Constant : Constant  Value=2*pi
  Demux : Demux  Outputs=2
  Math Function : Math  Operator=square  SaturateOnIntegerOverflow=on
  Math Function1 : Math  Operator=square  SaturateOnIntegerOverflow=on
  Math Function2 : Math  Operator=mod  SaturateOnIntegerOverflow=on
  Mux1 : Mux  Inputs=2
  Sqrt : Sqrt  SaturateOnIntegerOverflow=on
  Trigonometric Function : Trigonometry  Operator=atan2
  Polar [m,rad] : Outport
  wires:
  Add1/1 -> Demux/1
  Position 2 [m]/1 -> Add1/2
  Position 1 [m]/1 -> Add1/1
  Constant/1 -> Math Function2/2
  Math Function2/1 -> Mux1/2
  Bias/1 -> Math Function2/1
  Trigonometric Function/1 -> Bias/1
  Sqrt/1 -> Mux1/1
  Demux/2 -> Trigonometric Function/1, Math Function1/1
  Demux/1 -> Trigonometric Function/2, Math Function/1
  Math Function1/1 -> Add/2
  Math Function/1 -> Add/1
  Add/1 -> Sqrt/1
  Mux1/1 -> Polar [m,rad]/1

== system SqaureKF/Circuit/Rotate coordinates6 ==
  Position 1 [m] : Inport
  Position 2 [m] : Inport  Port=2
  Add : Sum
  Add1 : Sum  Inputs=+-
  Bias : Bias  Bias=2*pi
  Constant : Constant  Value=2*pi
  Demux : Demux  Outputs=2
  Math Function : Math  Operator=square  SaturateOnIntegerOverflow=on
  Math Function1 : Math  Operator=square  SaturateOnIntegerOverflow=on
  Math Function2 : Math  Operator=mod  SaturateOnIntegerOverflow=on
  Mux1 : Mux  Inputs=2
  Sqrt : Sqrt  SaturateOnIntegerOverflow=on
  Trigonometric Function : Trigonometry  Operator=atan2
  Polar [m,rad] : Outport
  wires:
  Mux1/1 -> Polar [m,rad]/1
  Add/1 -> Sqrt/1
  Math Function/1 -> Add/1
  Math Function1/1 -> Add/2
  Demux/1 -> Math Function/1, Trigonometric Function/2
  Demux/2 -> Math Function1/1, Trigonometric Function/1
  Sqrt/1 -> Mux1/1
  Trigonometric Function/1 -> Bias/1
  Bias/1 -> Math Function2/1
  Math Function2/1 -> Mux1/2
  Constant/1 -> Math Function2/2
  Position 1 [m]/1 -> Add1/1
  Position 2 [m]/1 -> Add1/2
  Add1/1 -> Demux/1

== system SqaureKF/Circuit/Rotate coordinates7 ==
  Position 1 [m] : Inport
  Position 2 [m] : Inport  Port=2
  Add : Sum
  Add1 : Sum  Inputs=+-
  Bias : Bias  Bias=2*pi
  Constant : Constant  Value=2*pi
  Demux : Demux  Outputs=2
  Math Function : Math  Operator=square  SaturateOnIntegerOverflow=on
  Math Function1 : Math  Operator=square  SaturateOnIntegerOverflow=on
  Math Function2 : Math  Operator=mod  SaturateOnIntegerOverflow=on
  Mux1 : Mux  Inputs=2
  Sqrt : Sqrt  SaturateOnIntegerOverflow=on
  Trigonometric Function : Trigonometry  Operator=atan2
  Polar [m,rad] : Outport
  wires:
  Add1/1 -> Demux/1
  Position 2 [m]/1 -> Add1/2
  Position 1 [m]/1 -> Add1/1
  Constant/1 -> Math Function2/2
  Math Function2/1 -> Mux1/2
  Bias/1 -> Math Function2/1
  Trigonometric Function/1 -> Bias/1
  Sqrt/1 -> Mux1/1
  Demux/2 -> Trigonometric Function/1, Math Function1/1
  Demux/1 -> Trigonometric Function/2, Math Function/1
  Math Function1/1 -> Add/2
  Math Function/1 -> Add/1
  Add/1 -> Sqrt/1
  Mux1/1 -> Polar [m,rad]/1

== system SqaureKF/Traffic/Heading Control ==
  Heading : Inport
  Heading Command : Inport  Port=2
  Derivative : Derivative
  Heading Error : Subsystem
  Integral : Subsystem  mask{Ki=0, Upper=1, Lower=-1}
      mask prompts: Ki "Gain"; Upper "Upper Limit"; Lower "Lower Limit"
  Kd : Gain  Gain=-0.2
  Kp : Gain  Gain=-0.5
  Reverse : Gain  Gain=-1
  Saturation : Saturate  UpperLimit=0.75  LowerLimit=-0.75
  Sum : Sum  Inputs=+++
  Roll Angle : Outport
  wires:
  Saturation/1 -> Roll Angle/1
  Reverse/1 -> Saturation/1
  Sum/1 -> Reverse/1
  Heading Error/1(Error) -> Integral/1(In1), Derivative/1, Kp/1
  Heading/1 -> Heading Error/1(Heading)
  Kp/1 -> Sum/2
  Integral/1(Out1) -> Sum/1
  Derivative/1 -> Kd/1
  Kd/1 -> Sum/3
  Heading Command/1 -> Heading Error/2(Command)

== system SqaureKF/Traffic/Height with Throttle ==
  Height : Inport
  Height  Command : Inport  Port=2
  Command3 : Constant  Value=0.5
  Derivative : Derivative
  Integral : Subsystem  mask{Ki=-0.001, Upper=1, Lower=-1}
      mask prompts: Ki "Gain"; Upper "Upper Limit"; Lower "Lower Limit"
  Kd : Gain  Gain=0
  Kp : Gain  Gain=-0.005
  Saturation : Saturate  UpperLimit=1  LowerLimit=0
  Sum : Sum  Inputs=+++
  Sum1 : Sum  Inputs=|+-
  Sum2 : Sum
  Throttle : Outport
  wires:
  Integral/1(Out1) -> Sum/1
  Command3/1 -> Sum2/2
  Sum/1 -> Sum2/1
  Sum2/1 -> Saturation/1
  Saturation/1 -> Throttle/1
  Sum1/1 -> Integral/1(In1), Derivative/1, Kp/1
  Height/1 -> Sum1/1
  Kp/1 -> Sum/2
  Derivative/1 -> Kd/1
  Kd/1 -> Sum/3
  Height  Command/1 -> Sum1/2

== system SqaureKF/Traffic/Speed with Pitch ==
  Speed : Inport
  Speed  Command : Inport  Port=2
  Derivative : Derivative
  Integral : Subsystem  mask{Ki=0.01, Upper=1, Lower=-1}
      mask prompts: Ki "Gain"; Upper "Upper Limit"; Lower "Lower Limit"
  Kd : Gain  Gain=0
  Kp : Gain  Gain=0.1
  Saturation : Saturate  UpperLimit=0.75  LowerLimit=-0.75
  Sum : Sum  Inputs=+++
  Sum1 : Sum  Inputs=|+-
  Pitch Angle : Outport
  wires:
  Speed  Command/1 -> Sum1/2
  Kd/1 -> Sum/3
  Derivative/1 -> Kd/1
  Integral/1(Out1) -> Sum/1
  Kp/1 -> Sum/2
  Speed/1 -> Sum1/1
  Sum1/1 -> Integral/1(In1), Kp/1, Derivative/1
  Sum/1 -> Saturation/1
  Saturation/1 -> Pitch Angle/1

== system SqaureKF/Traffic/Subsystem ==
  Vy : Inport
  Vx : Inport  Port=2
  Constant2 : Constant  Value=360
  Gain3 : Gain  Gain=180/pi
  Math Function1 : Math  Operator=mod  SaturateOnIntegerOverflow=on
  Trigonometric Function1 : Trigonometry  Operator=atan2
  trk : Outport
  wires:
  Trigonometric Function1/1 -> Gain3/1
  Constant2/1 -> Math Function1/2
  Gain3/1 -> Math Function1/1
  Math Function1/1 -> trk/1
  Vy/1 -> Trigonometric Function1/1
  Vx/1 -> Trigonometric Function1/2

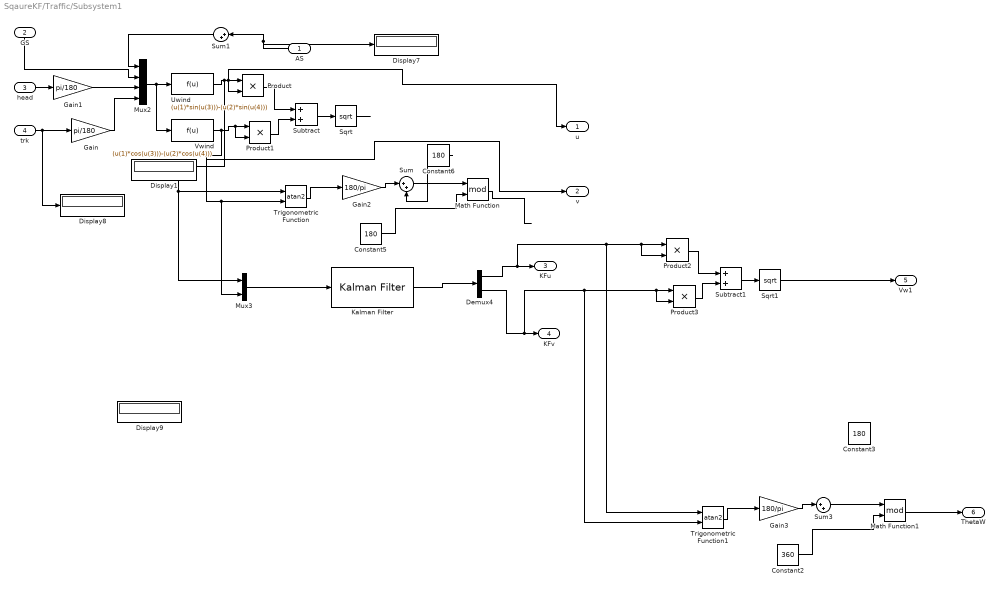
== system SqaureKF/Traffic/Subsystem1 ==
  AS : Inport
  GS : Inport  Port=2
  head : Inport  Port=3
  trk : Inport  Port=4
  Constant2 : Constant  Value=360
  Constant3 : Constant  Value=180
  Constant5 : Constant  Value=180
  Constant6 : Constant  Value=180
  Demux4 : Demux  Outputs=2
  Display{1,7..9} (4 alike) : Display
  Gain : Gain  Gain=pi/180
  Gain1 : Gain  Gain=pi/180
  Gain2 : Gain  Gain=180/pi
  Gain3 : Gain  Gain=180/pi
  Kalman Filter : dspadpt3/Kalman Filter  DialogController=dspDDGCreate  DialogControllerArgs=DataTag0  SystemSampleTime=-1  num_targets=1  sourceEnable=Always  isReset=on  X=[0,0]'  P=eye(2)  A=eye(2)  sourceMeasure=Specify via Dialog  H=eye(2)  Q=0.2*eye(2)  R=1E6*eye(2)  isOutputEstMeasure=off  isOutputEstState=on  isOutputEstError=off  isOutputPrdMeasure=off  isOutputPrdState=off  isOutputPrdError=off
  Math Function : Math  Operator=mod  SaturateOnIntegerOverflow=on
  Math Function1 : Math  Operator=mod  SaturateOnIntegerOverflow=on
  Mux2 : Mux
  Mux3 : Mux  Inputs=2
  Product{,1..3} (4 alike) : Product  RndMeth=Zero
  Sqrt : Sqrt  SaturateOnIntegerOverflow=on
  Sqrt1 : Sqrt  SaturateOnIntegerOverflow=on
  Subtract : Sum
  Subtract1 : Sum
  Sum : Sum  Inputs=|++
  Sum1 : Sum  Inputs=|++
  Sum3 : Sum  Inputs=|++
  Trigonometric Function : Trigonometry  Operator=atan2
  Trigonometric Function1 : Trigonometry  Operator=atan2
  Uwind : Fcn  Expr=(u(1)*sin(u(3)))-(u(2)*sin(u(4)))
  Vwind : Fcn  Expr=(u(1)*cos(u(3)))-(u(2)*cos(u(4)))
  u : Outport
  v : Outport  Port=2
  KFu : Outport  Port=3
  KFv : Outport  Port=4
  Vw1 : Outport  Port=5
  ThetaW : Outport  Port=6
  wires:
  Mux2/1 -> Uwind/1, Vwind/1
  Gain/1 -> Mux2/4
  Uwind/1 -> Product/1, Product/2, u/1, Trigonometric Function/1, Mux3/1
  Vwind/1 -> Product1/1, Product1/2, Trigonometric Function/2, Mux3/2, v/1
  Product/1 -> Subtract/1
  Product1/1 -> Subtract/2
  Subtract/1 -> Sqrt/1
  Trigonometric Function/1 -> Gain2/1
  Constant5/1 -> Math Function/2
  Sum/1 -> Math Function/1
  Gain2/1 -> Sum/1
  Mux3/1 -> Kalman Filter/1
  trk/1 -> Gain/1, Display8/1
  Constant6/1 -> Sum/2
  Demux4/1 -> KFu/1, Product2/1, Product2/2, Trigonometric Function1/1
  Demux4/2 -> KFv/1, Product3/1, Product3/2, Trigonometric Function1/2
  GS/1 -> Mux2/2
  Kalman Filter/1 -> Demux4/1
  AS/1 -> Sum1/1, Display7/1
  Sum1/1 -> Mux2/1
  Sqrt/1 -> ?
  Math Function/1 -> ?
  Product2/1 -> Subtract1/1
  Product3/1 -> Subtract1/2
  Subtract1/1 -> Sqrt1/1
  Sqrt1/1 -> Vw1/1
  Trigonometric Function1/1 -> Gain3/1
  Constant2/1 -> Math Function1/2
  Sum3/1 -> Math Function1/1
  Gain3/1 -> Sum3/1
  Math Function1/1 -> ThetaW/1
  head/1 -> Gain1/1
  Gain1/1 -> Mux2/3

== system SqaureKF/Traffic/Heading Control/Heading Error ==
  Heading : Inport
  Command : Inport  Port=2
  Abs : Abs
  Bias : Bias  Bias=2*pi
  Gain : Gain  Gain=-1
  Gain1 : Gain  Gain=-1
  Gain3 : Gain  Gain=-1
  Sum3 : Sum  Inputs=|+-
  Switch : Switch
  Switch1 : Switch
  Switch2 : Switch  Threshold=pi
  Error : Outport
  wires:
  Switch2/1 -> Error/1
  Switch1/1 -> Switch2/3
  Switch/1 -> Switch2/1
  Gain1/1 -> Switch/3
  Gain3/1 -> Switch1/1
  Bias/1 -> Switch/1, Gain1/1
  Gain/1 -> Bias/1
  Abs/1 -> Gain3/1, Switch2/2, Switch1/3, Gain/1
  Sum3/1 -> Switch1/2, Switch/2, Abs/1
  Command/1 -> Sum3/2
  Heading/1 -> Sum3/1

== system SqaureKF/Traffic/Heading Control/Integral ==
  In1 : Inport
  Integrator : Integrator  ExternalReset=either  LimitOutput=on  UpperSaturationLimit=Upper  LowerSaturationLimit=Lower
  Ki : Gain  Gain=Ki
  Out1 : Outport
  wires:
  In1/1 -> Ki/1
  Integrator/1 -> Out1/1
  [Mode] -> Integrator/2
  Ki/1 -> Integrator/1

== system SqaureKF/Traffic/Height with Throttle/Integral ==
  In1 : Inport
  Integrator : Integrator  ExternalReset=either  LimitOutput=on  UpperSaturationLimit=Upper  LowerSaturationLimit=Lower
  Ki : Gain  Gain=Ki
  Out1 : Outport
  wires:
  Ki/1 -> Integrator/1
  [Mode] -> Integrator/2
  Integrator/1 -> Out1/1
  In1/1 -> Ki/1

== system SqaureKF/Traffic/Speed with Pitch/Integral ==
  In1 : Inport
  Integrator : Integrator  ExternalReset=either  LimitOutput=on  UpperSaturationLimit=Upper  LowerSaturationLimit=Lower
  Ki : Gain  Gain=Ki
  Out1 : Outport
  wires:
  Ki/1 -> Integrator/1
  [Mode] -> Integrator/2
  Integrator/1 -> Out1/1
  In1/1 -> Ki/1

== matlab function Circuit/Embedded MATLAB Function ==
  data: d1 input double; i output double; d2 input double; d3 input double; d4 input double
function i = fcn(d1, d2, d3, d4)
%#eml

persistent j;

if isempty(j)
    j = 1;
end

%d = 40; 
v = 12;
vw =5;
omega = 0.38;
theta = pi/2;
d = v/omega * tan(theta/2);
d_upwind = 30;%(v-vw/2)/omega * tan(theta/2);
d_downwind = 30;%(v+vw)/omega * tan(theta/2);


if j==1 && d1 < d_downwind %bodge factor for !90 turn
    j = j + 1;
end

if j==2 && d2 < d_downwind
    j = j + 1;
end

if j==3 && d3 < d_upwind
    j = j + 1;
end

if j==4 && d4 < d_upwind
    j = 1;
end

i = j;
